simulink model "eqprop"  (R2024b)
settings: Solver=VariableStepAuto  StartTime=0.0  StopTime=1000  RelTol=1e-3
settings Model: Creator=merlin  LastModifiedBy=merlin

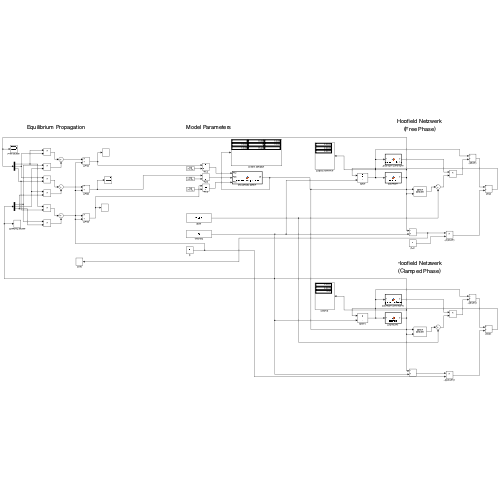
[thumbnail: Simulink's stored preview of the top-level diagram]
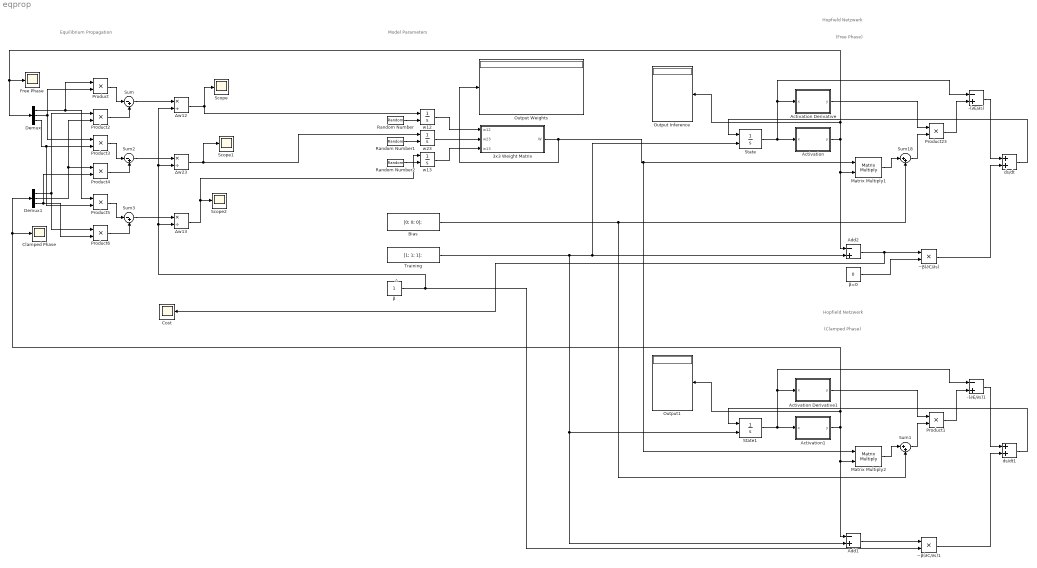
== system eqprop ==
  note: Δ
  note: Hopfield Netzwerk
  note: Equilibrium Propagation
  note: Model Parameters
  note: (Free Phase)
  note: (Clamped Phase)
  note: Hopfield Netzwerk
  -(∂E/∂s) : Sum  Inputs=-+
  -(∂E/∂s)1 : Sum  Inputs=-+
  3x3 Weight Matrix : MATLAB Function  TreatAsAtomicUnit=on
  Activation : MATLAB Function  TreatAsAtomicUnit=on
  Activation Derivative : MATLAB Function  TreatAsAtomicUnit=on
  Activation Derivative1 : MATLAB Function  TreatAsAtomicUnit=on
  Activation1 : MATLAB Function  TreatAsAtomicUnit=on
  Add1 : Sum  Inputs=-+
  Add2 : Sum  Inputs=-+
  Bias : Constant  Value=[0; 0; 0];  VectorParams1D=off
  Clamped Phase : Scope
  Cost : Scope
  Demux : Demux  Outputs=3
  Demux1 : Demux  Outputs=3
  Free Phase : Scope
  Matrix Multiply1 : Product  Multiplication=Matrix(*)
  Matrix Multiply2 : Product  Multiplication=Matrix(*)
  Output Inference : Display
  Output Weights : Display
  Output1 : Display
  Product{,1..6,23} (8 alike) : Product
  Random Number : RandomNumber  Seed=12  SampleTime=0.1
  Random Number1 : RandomNumber  Seed=23  SampleTime=0.1
  Random Number2 : RandomNumber  Seed=13  SampleTime=0.1
  Scope : Scope
  Scope1 : Scope
  Scope2 : Scope
  State : Integrator  InitialConditionSource=external
  State1 : Integrator  InitialConditionSource=external
  Sum : Sum  Inputs=|-+
  Sum1 : Sum  Inputs=|++
  Sum18 : Sum  Inputs=|++
  Sum2 : Sum  Inputs=|-+
  Sum3 : Sum  Inputs=|-+
  Training : Constant  Value=[1; 1; 1];  VectorParams1D=off
  ds/dt : Sum
  ds/dt1 : Sum
  w12 : Integrator  InitialConditionSource=external
  w13 : Integrator  InitialConditionSource=external
  w23 : Integrator  InitialConditionSource=external
  Δw12 : Product  Inputs=*/
  Δw13 : Product  Inputs=*/
  Δw23 : Product  Inputs=*/
  β : Constant
  β=0 : Constant  Value=0
  −β(∂C/∂s) : Product
  −β(∂C/∂s)1 : Product
  wires:
  State/1 -> -(∂E/∂s)/1, Activation Derivative/1(x), Activation/1(x)
  Activation Derivative/1(y) -> Product23/1
  Matrix Multiply1/1 -> Sum18/1
  ds/dt/1 -> State/1
  Activation/1(y) -> Matrix Multiply1/2, Add2/1, Free Phase/1, Demux/1, Output Inference/1
  -(∂E/∂s)/1 -> ds/dt/1
  −β(∂C/∂s)/1 -> ds/dt/2
  Add2/1 -> Cost/1, −β(∂C/∂s)/1
  Product23/1 -> -(∂E/∂s)/2
  Sum18/1 -> Product23/2
  Activation1/1(y) -> Matrix Multiply2/2, Add1/1, Demux1/1, Clamped Phase/1, Output1/1
  -(∂E/∂s)1/1 -> ds/dt1/1
  Matrix Multiply2/1 -> Sum1/1
  Add1/1 -> −β(∂C/∂s)1/1
  −β(∂C/∂s)1/1 -> ds/dt1/2
  Product1/1 -> -(∂E/∂s)1/2
  Activation Derivative1/1(y) -> Product1/1
  Sum1/1 -> Product1/2
  ds/dt1/1 -> State1/1
  State1/1 -> -(∂E/∂s)1/1, Activation Derivative1/1(x), Activation1/1(x)
  3x3 Weight Matrix/1(W) -> Output Weights/1, Matrix Multiply2/1, Matrix Multiply1/1
  Bias/1 -> Sum1/2, Sum18/2
  Training/1 -> Add1/2, State1/2, Add2/2, State/2
  β=0/1 -> −β(∂C/∂s)/2
  β/1 -> Δw13/2, Δw23/2, Δw12/2, −β(∂C/∂s)1/2
  Demux/1 -> Product5/1, Product/1
  Product/1 -> Sum/1
  Sum/1 -> Δw12/1
  Demux/2 -> Product/2, Product3/1
  Demux1/1 -> Product6/1, Product2/1
  Demux1/2 -> Product4/1, Product2/2
  Product2/1 -> Sum/2
  Δw12/1 -> Scope/1, w12/1
  Demux/3 -> Product5/2, Product3/2
  Product3/1 -> Sum2/1
  Demux1/3 -> Product6/2, Product4/2
  Product4/1 -> Sum2/2
  Sum2/1 -> Δw23/1
  Product5/1 -> Sum3/1
  Product6/1 -> Sum3/2
  Sum3/1 -> Δw13/1
  Δw23/1 -> w23/1, Scope1/1
  Δw13/1 -> w13/1, Scope2/1
  Random Number/1 -> w12/2
  Random Number1/1 -> w23/2
  Random Number2/1 -> w13/2
  w12/1 -> 3x3 Weight Matrix/1(w12)
  w23/1 -> 3x3 Weight Matrix/2(w23)
  w13/1 -> 3x3 Weight Matrix/3(w13)

== matlab function eqprop/3x3 Weight Matrix ==
  data: w12 input; w23 input; W output; w13 input
function W = create3x3WeightMatrix(w12, w23, w13)
    W = [0,    w12,  w13;
         w12,  0,    w23;
         w13,  w23,  0];
end

== matlab function eqprop/Activation1 ==
  data: x input; y output
function y = sigmoid(x)
y = 1 ./ (1 + exp(-x));
end

== matlab function eqprop/Activation Derivative ==
  data: x input; y output
function y = sigmoid_derivative(x)
sigmoid = 1 ./ (1 + exp(-x));
y = sigmoid .* (1 - sigmoid);
end

== matlab function eqprop/Activation ==
  data: x input; y output
function y = sigmoid(x)
y = 1 ./ (1 + exp(-x));
end

== matlab function eqprop/Activation Derivative1 ==
  data: x input; y output
function y = sigmoid_derivative(x)
sigmoid = 1 ./ (1 + exp(-x));
y = sigmoid .* (1 - sigmoid);
end
